simulink model "encoder_sensor"  (R2023a)
settings: configuration reference "config" (kept outside this file)
libraries: servo_hub_lib x1
settings Model: DataDictionary=model_config.sldd  Creator=hc  LastModifiedBy=Administrator
settings ConfigSetRef: SourceName=config

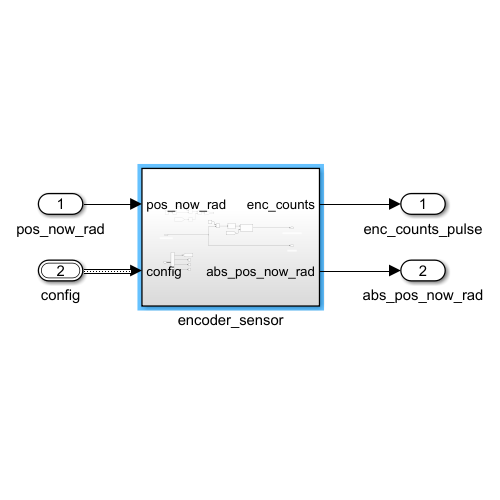
[thumbnail: Simulink's stored preview of the top-level diagram]
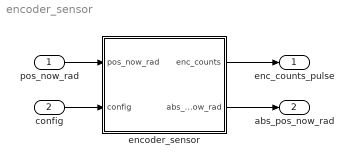
== system encoder_sensor ==
  pos_now_rad : Inport
  config : Inport  Port=2  OutDataTypeStr=Bus: SimPlantConfig  BusOutputAsStruct=on
  encoder_sensor : Subsystem
  enc_counts_pulse : Outport
  abs_pos_now_rad : Outport  Port=2
  wires:
  pos_now_rad/1 -> encoder_sensor/1(pos_now_rad)
  encoder_sensor/2(abs_pos_now_rad) -> abs_pos_now_rad/1
  encoder_sensor/1(enc_counts) -> enc_counts_pulse/1
  config/1 -> encoder_sensor/2(config)

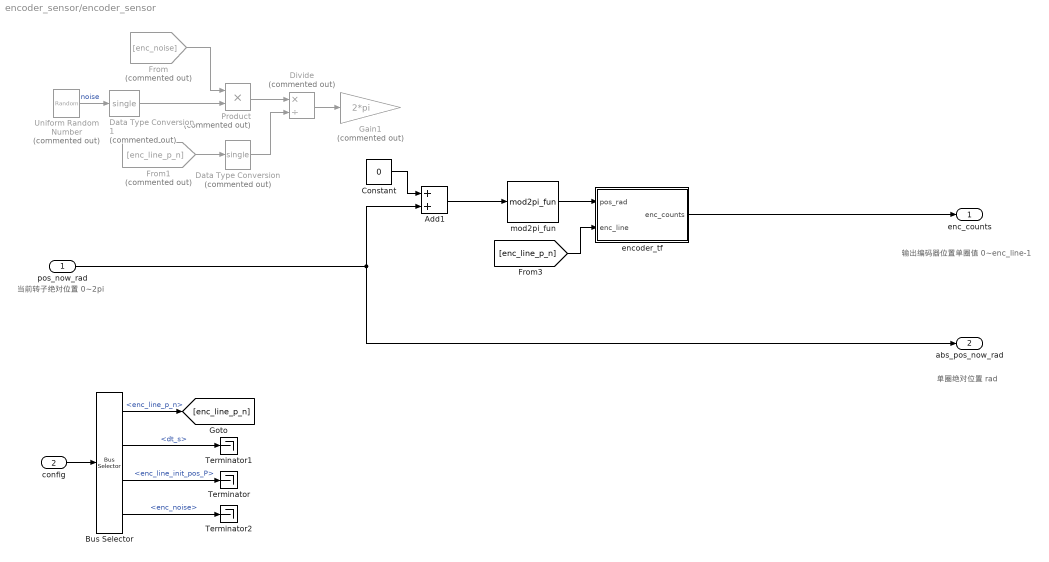
== system encoder_sensor/encoder_sensor ==
  note: 当前转子绝对位置 0~2pi
  note: 单圈绝对位置 rad
  note: 输出编码器位置单圈值 0~enc_line-1
  pos_now_rad : Inport
  config : Inport  Port=2
  Add1 : Sum
  Bus Selector : BusSelector  OutputSignals=enc_line_p_n,dt_s,enc_line_init_pos_P,enc_noise
  Constant : Constant  Value=0  OutDataTypeStr=single
  Data Type Conversion : DataTypeConversion  Commented=on  OutDataTypeStr=single  SaturateOnIntegerOverflow=off  RndMeth=Floor
  Data Type Conversion1 : DataTypeConversion  Commented=on  OutDataTypeStr=single  SaturateOnIntegerOverflow=off  RndMeth=Floor
  Divide : Product  Commented=on  Inputs=*/
  From : From  Commented=on  GotoTag=enc_noise
  From1 : From  Commented=on  GotoTag=enc_line_p_n
  Gain1 : Gain  Commented=on  Gain=2*pi
  Product : Product  Commented=on
  Terminator : Terminator
  Terminator1 : Terminator
  Terminator2 : Terminator
  Uniform Random Number : UniformRandomNumber  Commented=on  SampleTime=1e-5
  encoder_tf : Subsystem
  mod2pi_fun : servo_hub_lib/fast_math/mod2pi_fun  SystemSampleTime=-1  VariantActivationTime=update diagram  Latency=0  AutoFrameSizeCalculation=off
      settings: LibrarySourceBlock=|
      | simulink/User-Defined
      | Functions/MATLAB Function
  enc_counts : Outport
  abs_pos_now_rad : Outport  Port=2
  wires:
  Data Type Conversion1/1 -> Product/2
  Uniform Random Number/1 -> Data Type Conversion1/1  "noise"
  encoder_tf/1(enc_counts) -> enc_counts/1
  Add1/1 -> mod2pi_fun/1
  mod2pi_fun/1 -> encoder_tf/1(pos_rad)
  pos_now_rad/1 -> Add1/2, abs_pos_now_rad/1
  Product/1 -> Divide/1
  From1/1 -> Data Type Conversion/1
  Divide/1 -> Gain1/1
  config/1 -> Bus Selector/1
  Bus Selector/1 -> [enc_line_p_n]  "<enc_line_p_n>"
  Bus Selector/2 -> Terminator1/1  "<dt_s>"
  Bus Selector/3 -> Terminator/1  "<enc_line_init_pos_P>"
  Bus Selector/4 -> Terminator2/1  "<enc_noise>"
  From/1 -> Product/1
  [enc_line_p_n] -> encoder_tf/2(enc_line)
  Data Type Conversion/1 -> Divide/2
  Constant/1 -> Add1/1

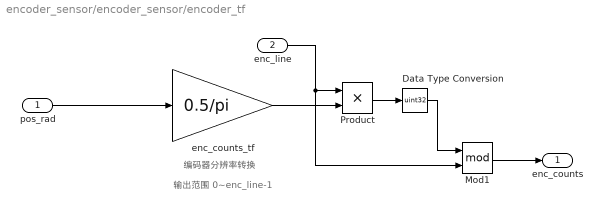
== system encoder_sensor/encoder_sensor/encoder_tf ==
  note: 输出范围 0~enc_line-1
  note: 编码器分辨率转换
  pos_rad : Inport  OutDataTypeStr=single
  enc_line : Inport  Port=2
  Data Type Conversion : DataTypeConversion  OutDataTypeStr=uint32  SaturateOnIntegerOverflow=off  RndMeth=Floor
  Mod1 : Math  Operator=mod
  Product : Product
  enc_counts_tf : Gain  Gain=0.5/pi
  enc_counts : Outport
  wires:
  enc_counts_tf/1 -> Product/2
  pos_rad/1 -> enc_counts_tf/1
  enc_line/1 -> Mod1/2, Product/1
  Mod1/1 -> enc_counts/1
  Product/1 -> Data Type Conversion/1
  Data Type Conversion/1 -> Mod1/1
